simulink model "PlantaCPDj"  (R2016b)
settings: Solver=VariableStepAuto  StartTime=0.0  StopTime=20  RelTol=1e-3
values from neighbouring files (symbols this model uses):
  kd = 2*wn*J-B    (= 4.82)    [hurwitz.m]
  kp = wn^2*J    (= 21.6)    [hurwitz.m]
settings Model: Creator=Dell  LastModifiedBy=Dell

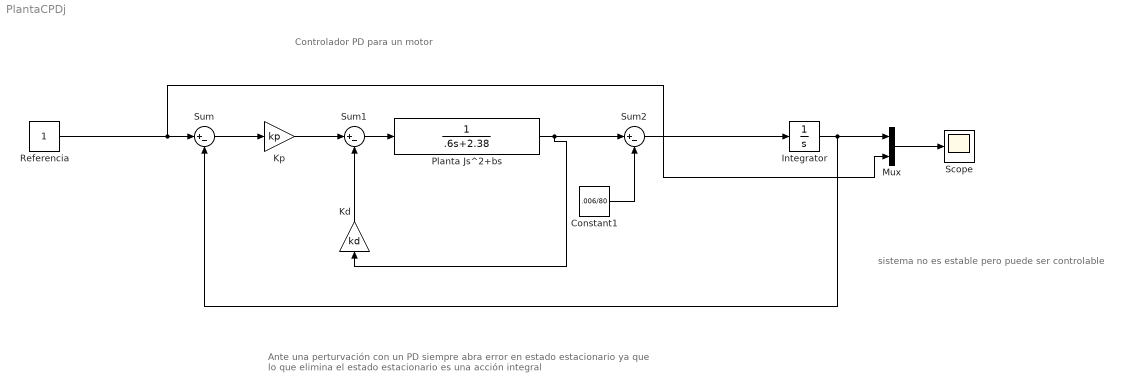
== system PlantaCPDj ==
  note: sistema no es estable pero puede ser controlable
  note: Controlador PD para un motor
  note: Ante una perturvación con un PD  siempre abra error en estado estacionario
      | ya que lo que elimina el estado estacionario es una acción integral
  Constant1 : Constant  Value=.006/80
  Integrator : Integrator
  Kd : Gain  Gain=kd
  Kp : Gain  Gain=kp
  Mux : Mux  Inputs=2
  Planta Js^2+bs : TransferFcn  Denominator=[.6 2.38 ]
  Referencia : Constant
  Scope : Scope
  Sum : Sum  Inputs=|+-
  Sum1 : Sum  Inputs=|+-
  Sum2 : Sum  Inputs=|+-
  wires:
  Kp/1 -> Sum1/1
  Sum/1 -> Kp/1
  Sum1/1 -> Planta Js^2+bs/1
  Kd/1 -> Sum1/2
  Planta Js^2+bs/1 -> Sum2/1, Kd/1
  Integrator/1 -> Mux/1, Sum/2
  Referencia/1 -> Mux/2, Sum/1
  Mux/1 -> Scope/1
  Sum2/1 -> Integrator/1
  Constant1/1 -> Sum2/2
